simulink model "myRegression2In2Mid1Out"  (R2024a)
settings: Solver=VariableStepAuto  StartTime=0.0  StopTime=10.0  RelTol=1e-3
InitFcn:
  | close all;
  | clear all;
  | % 入力格子（行列）作成
  | [x1, x2] = meshgrid(-1.2:0.1:1.2, -1.2:0.1:1.2);
  | y = zeros(10, 10);
StopFcn:
  | y = out.y.Data;
  | surf(x1, x2, y);
  | colorbar;
undefined symbols (not defined in the file or in its folder): x1, x2
libraries: neural x3
settings Model: Creator=mashi  LastModifiedBy=mashi

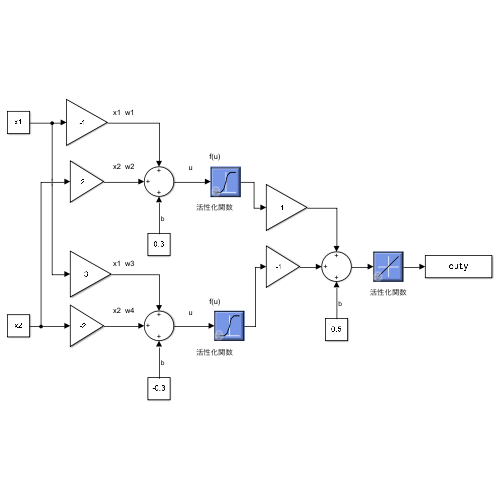
[thumbnail: Simulink's stored preview of the top-level diagram]
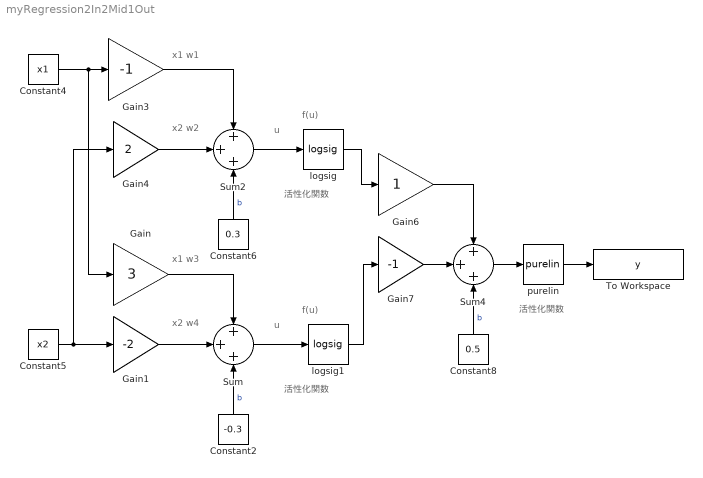
== system myRegression2In2Mid1Out ==
  note: 活性化関数
  note: u
  note: f(u)
  note: x2 w4
  note: x1 w3
  note: 活性化関数
  note: u
  note: f(u)
  note: x2 w2
  note: x1 w1
  note: 活性化関数
  Constant2 : Constant  Value=-0.3
  Constant4 : Constant  Value=x1
  Constant5 : Constant  Value=x2
  Constant6 : Constant  Value=0.3
  Constant8 : Constant  Value=0.5
  Gain : Gain  Gain=3
  Gain1 : Gain  Gain=-2
  Gain3 : Gain  Gain=-1
  Gain4 : Gain  Gain=2
  Gain6 : Gain
  Gain7 : Gain  Gain=-1
  Sum : Sum  Inputs=+++
  Sum2 : Sum  Inputs=+++
  Sum4 : Sum  Inputs=+++
  To Workspace : ToWorkspace  VariableName=y  SaveFormat=Timeseries  SampleTime=-1
  logsig : neural/Transfer Functions/logsig
  logsig1 : neural/Transfer Functions/logsig
  purelin : neural/Transfer Functions/purelin
  wires:
  Gain/1 -> Sum/1
  Gain1/1 -> Sum/2
  Constant2/1 -> Sum/3  "b"
  Constant6/1 -> Sum2/3  "b"
  Gain4/1 -> Sum2/2
  Gain3/1 -> Sum2/1
  Constant4/1 -> Gain/1, Gain3/1
  Constant8/1 -> Sum4/3  "b"
  Sum4/1 -> purelin/1
  Gain7/1 -> Sum4/2
  Gain6/1 -> Sum4/1
  Constant5/1 -> Gain4/1, Gain1/1
  Sum2/1 -> logsig/1
  logsig/1 -> Gain6/1
  Sum/1 -> logsig1/1
  logsig1/1 -> Gain7/1
  purelin/1 -> To Workspace/1
